simulink model "torqueBalancing2012b"  (Simulink 8.0)
settings: Solver=FixedStepDiscrete  StartTime=0.0  StopTime=CONFIG.SIMULATION_TIME  FixedStep=CONFIG.Ts  RelTol=1e-3
InitFcn:
  | initTorqueBalancing;
values from neighbouring files (symbols this model uses):
  baseToWorldRotationPort = ['/' WBT_modelName '/floatingBaseRotationMatrix:i']    [initTorqueBalancing.m]
  WBT_modelName = 'matlabTorqueBalancing'    [initTorqueBalancing.m]
undefined symbols (not defined in the file or in its folder): bVectorConstraints, CONFIG, ConstraintsMatrix, DiscIntNeverNeededParam, gain, impedencesSat, reg, ROBOT_DOF, ROBOT_DOF_FOR_SIMULINK, sat, SM, sm, Ts
libraries: WBToolboxLibrary x139, simulink x11, WBCLibrary x2
(part 1 of 3)
settings Model: Creator=daniele  LastModifiedBy=gnava
settings DebuggingCC: FcnCallInpInsideContextMsg=EnableAllAsWarning  FrameProcessingCompatibilityMsg=error
settings SFSimCC: SimParseCustomCode=off
settings CodeAppCC: CustomSymbolStrType=$N$R$M_T
settings GRTTargetCC: CodeReplacementLibrary=C89/C90 (ANSI)  CombineOutputUpdateFcns=off  GRTInterface=on

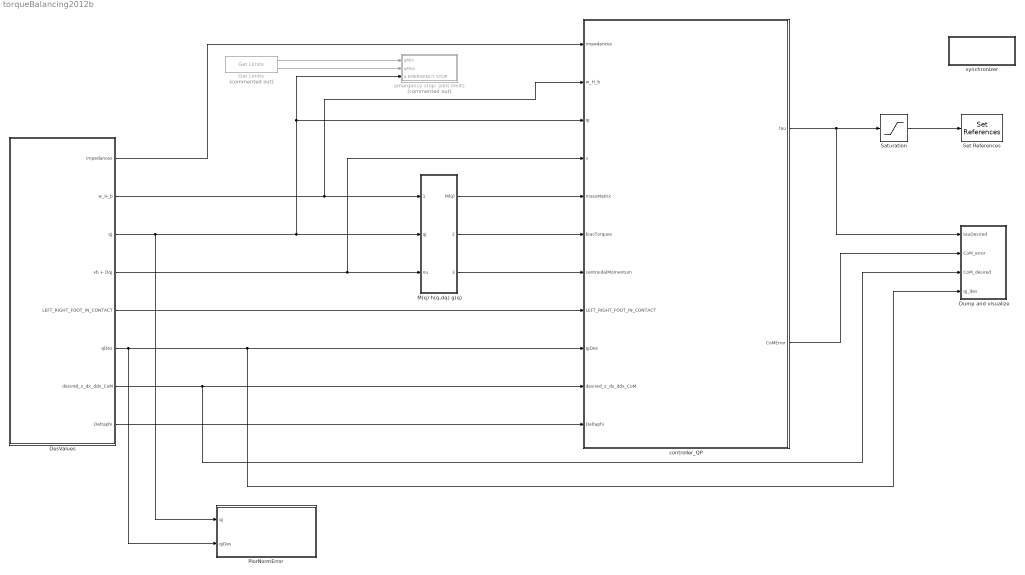
== system torqueBalancing2012b ==
  DesValues : Subsystem  Priority=-10
  Dump and visualize : Subsystem
  Get Limits : WBToolboxLibrary/wholeBodyStates/Get Limits  Commented=on  limitsType=Position  robotName=WBT_robotName  localName=WBT_modelName  wbiFile=WBT_wbiFilename  wbiList=WBT_wbiList
  M(q) h(q,dq) g(q) : Subsystem
  PlorNormError : Subsystem
  Saturation : Saturate  UpperLimit=sat.torque  LowerLimit=-sat.torque
  Set References : WBToolboxLibrary/wholeBodyActuators/Set References  controlType=Torque  robotName=WBT_robotName  localName=WBT_modelName  wbiFile=WBT_wbiFilename  wbiList=WBT_wbiList
  controller_QP : Subsystem
  emergency stop: joint limits : Subsystem  Commented=on
  synchronizer : Subsystem
      mask Display: disp('SYNCHRONIZER')
  wires:
  M(q) h(q,dq) g(q)/1(M(q)) -> controller_QP/5(massMatrix)
  Get Limits/1 -> emergency stop: joint limits/1(qMin)
  Get Limits/2 -> emergency stop: joint limits/2(qMax)
  M(q) h(q,dq) g(q)/2(biasTorques) -> controller_QP/6(biasTorques)
  M(q) h(q,dq) g(q)/3(H(q,dq)) -> controller_QP/7(centroidalMomentum)
  controller_QP/1("tau ") -> Dump and visualize/1(tauDesired), Saturation/1
  controller_QP/2(CoMError) -> Dump and visualize/2(CoM_error)
  DesValues/6(qDes) -> PlorNormError/2(qjDes), controller_QP/9(qjDes), Dump and visualize/4(qj_des)
  DesValues/5(LEFT_RIGHT_FOOT_IN_CONTACT) -> controller_QP/8(LEFT_RIGHT_FOOT_IN_CONTACT)
  DesValues/7(desired_x_dx_ddx_CoM) -> Dump and visualize/3(CoM_desired), controller_QP/10(desired_x_dx_ddx_CoM)
  DesValues/1(impedances) -> controller_QP/1(impedances)
  Saturation/1 -> Set References/1
  DesValues/2(w_H_b) -> controller_QP/2(w_H_b), M(q) h(q,dq) g(q)/1(w_H_b)
  DesValues/4(vb + Dqj) -> controller_QP/4(v), M(q) h(q,dq) g(q)/3(nu)
  DesValues/3(qj) -> PlorNormError/1(qj), emergency stop: joint limits/3(q EMERGENCY STOP), controller_QP/3(qj), M(q) h(q,dq) g(q)/2(qj)
  DesValues/8(Deltaphi) -> controller_QP/11(Deltaphi)

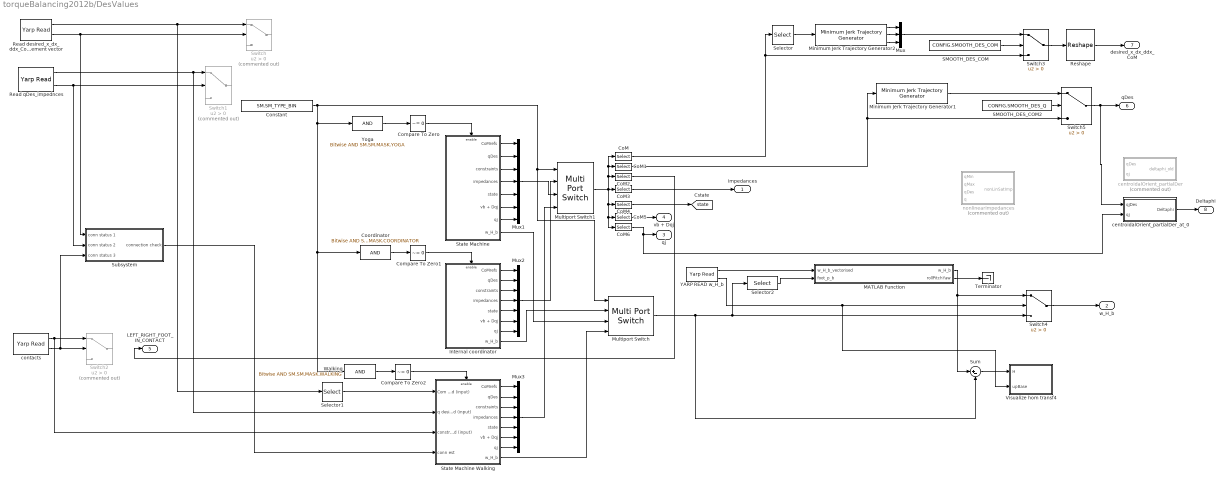
== system torqueBalancing2012b/DesValues ==
  CoM : Selector  InputPortWidth=18+4*ROBOT_DOF  IndexOptions=Index vector (dialog)  Indices=[1:9]  OutputSizes=1
  CoM1 : Selector  InputPortWidth=18+4*ROBOT_DOF  IndexOptions=Index vector (dialog)  Indices=[10:9+ROBOT_DOF]  OutputSizes=1
  CoM2 : Selector  InputPortWidth=18+4*ROBOT_DOF  IndexOptions=Index vector (dialog)  Indices=[10+ROBOT_DOF,11+ROBOT_DOF]  OutputSizes=1
  CoM3 : Selector  InputPortWidth=18+4*ROBOT_DOF  IndexOptions=Index vector (dialog)  Indices=[12+ROBOT_DOF:11+2*ROBOT_DOF]  OutputSizes=1
  CoM4 : Selector  InputPortWidth=18+4*ROBOT_DOF  IndexOptions=Index vector (dialog)  Indices=[12+2*ROBOT_DOF]  OutputSizes=1
  CoM5 : Selector  InputPortWidth=18+4*ROBOT_DOF  IndexOptions=Index vector (dialog)  Indices=[13+2*ROBOT_DOF:18+3*ROBOT_DOF]  OutputSizes=1
  CoM6 : Selector  InputPortWidth=18+4*ROBOT_DOF  IndexOptions=Index vector (dialog)  Indices=[19+3*ROBOT_DOF:18+4*ROBOT_DOF]  OutputSizes=1
  Compare To Zero : simulink/Logic and Bit Operations/Compare To Zero  relop=~=  OutDataTypeStr=boolean
  Compare To Zero1 : simulink/Logic and Bit Operations/Compare To Zero  relop=~=  OutDataTypeStr=boolean
  Compare To Zero2 : simulink/Logic and Bit Operations/Compare To Zero  relop=~=  OutDataTypeStr=boolean
  Constant : Constant  Priority=-10  Value=SM.SM_TYPE_BIN  OutDataTypeStr=uint8
  Coordinator : simulink/Logic and Bit Operations/Bitwise Operator  logicop=AND  UseBitMask=on  BitMask=SM.SM.MASK.COORDINATOR  BitMaskRealWorld=Stored Integer
  Internal coordinator : Subsystem
  MATLAB Function : MATLAB Function  TreatAsAtomicUnit=on
  Minimum Jerk Trajectory Generator1 : WBToolboxLibrary/Utilities/Minimum Jerk Trajectory Generator  externalSettlingTime=off  settlingTime=references.joints.smoothingTime  sampleTime=CONFIG.Ts  firstDerivatives=off  secondDerivatives=off  explicitInitialValue=off
  Minimum Jerk Trajectory Generator2 : WBToolboxLibrary/Utilities/Minimum Jerk Trajectory Generator  externalSettlingTime=off  settlingTime=references.com.smoothingTime  sampleTime=CONFIG.Ts  firstDerivatives=on  secondDerivatives=on  explicitInitialValue=off
  Multiport Switch : MultiPortSwitch  DataPortOrder=Specify indices  DataPortIndices={1, 2, 4}
  Multiport Switch1 : MultiPortSwitch  DataPortOrder=Specify indices  DataPortIndices={1, 2, 4}
  Mux : Mux  Inputs=3
  Mux1 : Mux  Inputs=7
  Mux2 : Mux  Inputs=7
  Mux3 : Mux  Inputs=7
  Read desired_x_dx_ddx_CoM as 9 element vector : WBToolboxLibrary/Utilities/Yarp Read  portName=['/' WBT_modelName '/comDes:i']  signalSize=9  blocking=off  timestamp=off  autoconnect=off  errorOnConnection=on
  Read qDes_impednces : WBToolboxLibrary/Utilities/Yarp Read  portName=['/' WBT_modelName '/qDes:i']  signalSize=ROBOT_DOF  blocking=off  timestamp=off  autoconnect=off  errorOnConnection=on
  Reshape : Reshape  OutputDimensionality=Customize  OutputDimensions=[3,3]
  SMOOTH_DES_COM : Constant  Value=CONFIG.SMOOTH_DES_COM
  SMOOTH_DES_COM2 : Constant  Value=CONFIG.SMOOTH_DES_Q
  Selector : Selector  InputPortWidth=9  IndexOptions=Index vector (dialog)  Indices=[1 2 3]  OutputSizes=1
  Selector1 : Selector  InputPortWidth=9  IndexOptions=Index vector (dialog)  Indices=[1 2 3]  OutputSizes=1
  Selector2 : Selector  NumberOfDimensions=2  InputPortWidth=3  IndexOptions=Index vector (dialog),Index vector (dialog)  Indices=[1 2 3],4  OutputSizes=1,1
  State Machine : Subsystem  Priority=-100
  State Machine Walking : Subsystem  Priority=-100
  Subsystem : Subsystem
  Sum : Sum  Inputs=|+-
  Switch : Switch  Commented=on  Criteria=u2 > Threshold
  Switch1 : Switch  Commented=on  Criteria=u2 > Threshold
  Switch2 : Switch  Commented=on  Criteria=u2 > Threshold
  Switch3 : Switch  Criteria=u2 > Threshold
  Switch4 : Switch  Criteria=u2 > Threshold
  Switch5 : Switch  Criteria=u2 > Threshold
  Terminator : Terminator
  Visualize hom transf4 : Subsystem
  Walking : simulink/Logic and Bit Operations/Bitwise Operator  logicop=AND  UseBitMask=on  BitMask=SM.SM.MASK.WALKING  BitMaskRealWorld=Stored Integer
  YARP READ w_H_b : WBToolboxLibrary/Utilities/Yarp Read  portName=[baseToWorldRotationPort]  signalSize=16  blocking=off  timestamp=off  autoconnect=off  errorOnConnection=on
  Yoga : simulink/Logic and Bit Operations/Bitwise Operator  logicop=AND  UseBitMask=on  BitMask=SM.SM.MASK.YOGA  BitMaskRealWorld=Stored Integer
  centroidalOrient_partialDer : Subsystem  Commented=on
  centroidalOrient_partialDer_at_0 : Subsystem
  contacts : WBToolboxLibrary/Utilities/Yarp Read  portName=['/' WBT_modelName '/constraints:i']  signalSize=2  blocking=off  timestamp=off  autoconnect=off  errorOnConnection=on
  nonlinearImpedances : Subsystem  Commented=on
  impedances : Outport
  w_H_b : Outport  Port=2
  qj : Outport  Port=3
  vb + Dqj : Outport  Port=4
  LEFT_RIGHT_FOOT_IN_CONTACT : Outport  Port=5
  qDes : Outport  Port=6
  desired_x_dx_ddx_CoM : Outport  Port=7
  Deltaphi : Outport  Port=8
  tag scope: state=global
  wires:
  Read desired_x_dx_ddx_CoM as 9 element vector/2 -> Subsystem/1(conn status 1), Switch/2
  Read desired_x_dx_ddx_CoM as 9 element vector/1 -> Selector1/1, Switch/1
  Reshape/1 -> desired_x_dx_ddx_CoM/1
  Read qDes_impednces/2 -> Subsystem/2(conn status 2), Switch1/2
  contacts/2 -> Subsystem/3(conn status 3), Switch2/2
  CoM2/1 -> LEFT_RIGHT_FOOT_IN_CONTACT/1
  CoM/1 -> Selector/1, Switch3/3
  Selector/1 -> Minimum Jerk Trajectory Generator2/1
  Minimum Jerk Trajectory Generator2/1 -> Mux/1
  Minimum Jerk Trajectory Generator2/2 -> Mux/2
  Minimum Jerk Trajectory Generator2/3 -> Mux/3
  Mux/1 -> Switch3/1
  Switch3/1 -> Reshape/1
  SMOOTH_DES_COM/1 -> Switch3/2
  SMOOTH_DES_COM2/1 -> Switch5/2
  CoM1/1 -> Minimum Jerk Trajectory Generator1/1, Switch5/3
  Constant/1 -> Multiport Switch/1, Multiport Switch1/1, Coordinator/1, Walking/1, Yoga/1
  State Machine/3(constraints) -> Mux1/3
  State Machine/2(qDes) -> Mux1/2
  State Machine/1(CoMrefs) -> Mux1/1
  Internal coordinator/1(CoMrefs) -> Mux2/1
  Internal coordinator/2(qDes) -> Mux2/2
  Internal coordinator/3(constraints) -> Mux2/3
  Multiport Switch1/1 -> CoM/1, CoM1/1, CoM2/1, CoM6/1, CoM5/1, CoM4/1, CoM3/1
  CoM3/1 -> impedances/1
  State Machine/4(impedances) -> Mux1/4
  Internal coordinator/4(impedances) -> Mux2/4
  State Machine/5(state) -> Mux1/5
  Internal coordinator/5(state) -> Mux2/5
  CoM4/1 -> [state]
  Internal coordinator/6(vb + Dqj) -> Mux2/6
  Internal coordinator/7(qj) -> Mux2/7
  State Machine/6(vb + Dqj) -> Mux1/6
  State Machine/7(qj) -> Mux1/7
  CoM5/1 -> vb + Dqj/1
  Minimum Jerk Trajectory Generator1/1 -> Switch5/1
  State Machine Walking/4(impedances) -> Mux3/4
  State Machine Walking/3(constraints) -> Mux3/3
  State Machine Walking/5(state) -> Mux3/5
  State Machine Walking/6(vb + Dqj) -> Mux3/6
  State Machine Walking/1(CoMrefs) -> Mux3/1
  State Machine Walking/7(qj) -> Mux3/7
  Coordinator/1 -> Compare To Zero1/1
  Yoga/1 -> Compare To Zero/1
  Walking/1 -> Compare To Zero2/1
  Mux3/1 -> Multiport Switch1/4
  State Machine Walking/8(w_H_b) -> Multiport Switch/4
  Selector1/1 -> State Machine Walking/1(Com desired (input))
  Compare To Zero/1 -> State Machine/Enable
  Compare To Zero1/1 -> Internal coordinator/Enable
  Compare To Zero2/1 -> State Machine Walking/Enable
  Mux1/1 -> Multiport Switch1/3
  Mux2/1 -> Multiport Switch1/2
  State Machine/8(w_H_b) -> Multiport Switch/3
  Internal coordinator/8(w_H_b) -> Multiport Switch/2
  Read qDes_impednces/1 -> State Machine Walking/2(q desired (input)), Switch1/1
  Subsystem/1(connection check) -> State Machine Walking/4(conn est)
  State Machine Walking/2(qDes) -> Mux3/2
  contacts/1 -> State Machine Walking/3(constraints desired (input)), Switch2/1
  YARP READ w_H_b/1 -> MATLAB Function/1(w_H_b_vectorised)
  MATLAB Function/1(w_H_b) -> Sum/1, Switch4/1
  Selector2/1 -> MATLAB Function/2(foot_p_b)
  Sum/1 -> Visualize hom transf4/1(H)
  Switch4/1 -> w_H_b/1
  Multiport Switch/1 -> Selector2/1, Switch4/3, Sum/2
  YARP READ w_H_b/2 -> Switch4/2, Visualize hom transf4/2(upBase)
  MATLAB Function/2(rollPitchYaw) -> Terminator/1
  Switch5/1 -> centroidalOrient_partialDer_at_0/1(qjDes), qDes/1
  CoM6/1 -> centroidalOrient_partialDer_at_0/2(qj), qj/1
  centroidalOrient_partialDer_at_0/1(Deltaphi) -> Deltaphi/1

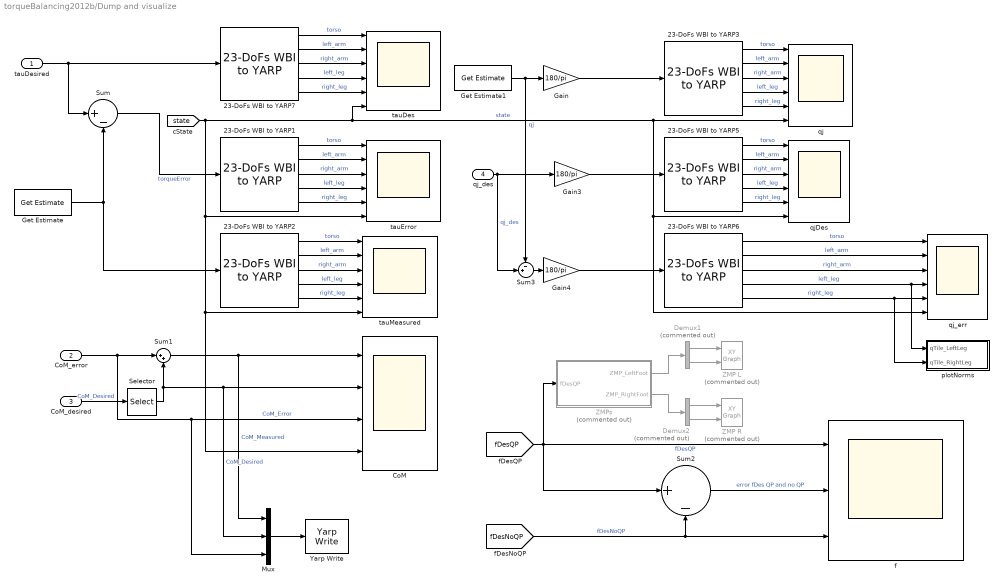
== system torqueBalancing2012b/Dump and visualize ==
  tauDesired : Inport
  CoM_error : Inport  Port=2
  CoM_desired : Inport  Port=3
  qj_des : Inport  Port=4
  23-DoFs WBI to YARP{1..3,5..7} (6 alike) : WBToolboxLibrary/Utilities/23-DoFs WBI to YARP
  CoM : Scope  NumInputPorts=4
      settings: ShowLegends=on  TimeRange=400  YMin=-0.22651~-0.2206~-0.01616~-0.125  YMax=0.64756~0.64126~0.01985~11.125  SaveName=CoM_data
  Demux1 : Demux  Commented=on  Outputs=2
  Demux2 : Demux  Commented=on  Outputs=2
  Gain : Gain  Gain=180/pi
  Gain3 : Gain  Gain=180/pi
  Gain4 : Gain  Gain=180/pi
  Get Estimate : WBToolboxLibrary/wholeBodyStates/Get Estimate  estimateType=Joints Torque  robotName=WBT_robotName  localName=WBT_modelName  wbiFile=WBT_wbiFilename  wbiList=WBT_wbiList
  Get Estimate1 : WBToolboxLibrary/wholeBodyStates/Get Estimate  estimateType=Joints Position  robotName=WBT_robotName  localName=WBT_modelName  wbiFile=WBT_wbiFilename  wbiList=WBT_wbiList
  Mux : Mux  Inputs=3
  Selector : Selector  NumberOfDimensions=2  IndexOptions=Index vector (dialog),Index vector (dialog)  Indices=[1:3],1  OutputSizes=1,1
  Sum : Sum  Inputs=|+-
  Sum1 : Sum  Inputs=|++
  Sum2 : Sum  Inputs=|+-
  Sum3 : Sum  Inputs=-+|
  Yarp Write : WBToolboxLibrary/Utilities/Yarp Write  portName='/oneFootBalancing/comInfo:o'  autoconnect=off  errorOnConnection=on
  ZMP L : simulink/Sinks/XY Graph  Commented=on  xmin=gain.footSize(1,1)  xmax=gain.footSize(1,2)  ymin=gain.footSize(2,1)  ymax=gain.footSize(2,2)  st=-1
  ZMP R : simulink/Sinks/XY Graph  Commented=on  xmin=gain.footSize(1,1)  xmax=gain.footSize(1,2)  ymin=gain.footSize(2,1)  ymax=gain.footSize(2,2)  st=-1
  ZMPs : Subsystem  Commented=on
  f : Scope  NumInputPorts=3
      settings: TimeRange=40  YMin=-57.20094~-0.00771~-57.19974  YMax=249.13374~0.00771~249.13391  SaveName=ScopeData2
  plotNorms : Subsystem
  qj : Scope  NumInputPorts=6
      settings: ShowLegends=on  TimeRange=40  YMin=-32.23366~-73.47113~-76.53021~-115.83931~-22.69232~-0.125  YMax=12.59592~104.84995~80.45225~96.1311~29.20641~11.125  SaveName=qj_and_v
  qjDes : Scope  NumInputPorts=6
      settings: ShowLegends=on  TimeRange=40  YMin=-3.5~-40~-40~-15~-10~2  YMax=0.5~50~50~15~12.5~2  SaveName=qj_and_v3
  qj_err : Scope  NumInputPorts=6
      settings: ShowLegends=on  TimeRange=40  YMin=-5~-3~-2~-7.5~-3~2  YMax=3~4~3.5~7.5~6~2  SaveName=qj_and_v4
  tauDes : Scope  NumInputPorts=6
      settings: ShowLegends=on  TimeRange=14  YMin=-58.64434~-21.39097~-21.52762~-81.43596~-94.54214~0.625  YMax=46.53013~21.42382~22.63023~161.15223~80.75083~4.375  SaveName=tauDes
  tauError : Scope  NumInputPorts=6
      settings: ShowLegends=on  TimeRange=90  YMin=-2.6459~-3.11955~-3.43578~-20.45507~-6.22161~0.625  YMax=3.57267~4.34787~4.22527~21.32013~5.56801~4.375  SaveName=tauError
  tauMeasured : Scope  NumInputPorts=6
      settings: ShowLegends=on  TimeRange=14  YMin=-7~-2.5~-2.5~-3~-4~2  YMax=0~1.5~1.5~2~3~2  SaveName=tauMeasured
  wires:
  CoM_error/1 -> Sum1/1, Mux/3, CoM/3  "CoM_Error"
  CoM_desired/1 -> Selector/1  "CoM_Desired"
  Sum1/1 -> Mux/1, CoM/1  "CoM_Measured"
  Get Estimate1/1 -> Sum3/1, Gain/1  "qj"
  Gain/1 -> 23-DoFs WBI to YARP3/1
  23-DoFs WBI to YARP3/5 -> qj/5  "right_leg"
  23-DoFs WBI to YARP3/1 -> qj/1  "torso"
  23-DoFs WBI to YARP3/2 -> qj/2  "left_arm"
  23-DoFs WBI to YARP3/4 -> qj/4  "left_leg"
  23-DoFs WBI to YARP3/3 -> qj/3  "right_arm"
  [fDesQP] -> ZMPs/1(fDesQP), Sum2/1, f/1  "fDesQP"
  ZMPs/1(ZMP_LeftFoot) -> Demux1/1
  ZMPs/2(ZMP_RightFoot) -> Demux2/1
  Demux1/1 -> ZMP L/1
  Demux1/2 -> ZMP L/2
  Demux2/1 -> ZMP R/1
  Demux2/2 -> ZMP R/2
  Sum2/1 -> f/2  "error fDes QP and no QP"
  [fDesNoQP] -> Sum2/2, f/3  "fDesNoQP"
  tauDesired/1 -> 23-DoFs WBI to YARP7/1, Sum/1
  Get Estimate/1 -> 23-DoFs WBI to YARP2/1, Sum/2
  23-DoFs WBI to YARP7/5 -> tauDes/5  "right_leg"
  23-DoFs WBI to YARP7/1 -> tauDes/1  "torso"
  23-DoFs WBI to YARP7/2 -> tauDes/2  "left_arm"
  23-DoFs WBI to YARP7/4 -> tauDes/4  "left_leg"
  23-DoFs WBI to YARP7/3 -> tauDes/3  "right_arm"
  23-DoFs WBI to YARP1/5 -> tauError/5  "right_leg"
  23-DoFs WBI to YARP1/1 -> tauError/1  "torso"
  23-DoFs WBI to YARP1/2 -> tauError/2  "left_arm"
  23-DoFs WBI to YARP1/4 -> tauError/4  "left_leg"
  23-DoFs WBI to YARP1/3 -> tauError/3  "right_arm"
  Sum/1 -> 23-DoFs WBI to YARP1/1  "torqueError"
  23-DoFs WBI to YARP2/5 -> tauMeasured/5  "right_leg"
  23-DoFs WBI to YARP2/1 -> tauMeasured/1  "torso"
  23-DoFs WBI to YARP2/2 -> tauMeasured/2  "left_arm"
  23-DoFs WBI to YARP2/4 -> tauMeasured/4  "left_leg"
  23-DoFs WBI to YARP2/3 -> tauMeasured/3  "right_arm"
  qj_des/1 -> Sum3/2, Gain3/1  "qj_des"
  Gain3/1 -> 23-DoFs WBI to YARP5/1
  23-DoFs WBI to YARP5/5 -> qjDes/5  "right_leg"
  23-DoFs WBI to YARP5/1 -> qjDes/1  "torso"
  23-DoFs WBI to YARP5/2 -> qjDes/2  "left_arm"
  23-DoFs WBI to YARP5/4 -> qjDes/4  "left_leg"
  23-DoFs WBI to YARP5/3 -> qjDes/3  "right_arm"
  Gain4/1 -> 23-DoFs WBI to YARP6/1
  23-DoFs WBI to YARP6/5 -> plotNorms/2(qTile_RightLeg), qj_err/5  "right_leg"
  23-DoFs WBI to YARP6/1 -> qj_err/1  "torso"
  23-DoFs WBI to YARP6/2 -> qj_err/2  "left_arm"
  23-DoFs WBI to YARP6/4 -> plotNorms/1(qTile_LeftLeg), qj_err/4  "left_leg"
  23-DoFs WBI to YARP6/3 -> qj_err/3  "right_arm"
  Sum3/1 -> Gain4/1
  Selector/1 -> Sum1/2, Mux/2, CoM/2  "CoM_Desired"
  [state] -> tauDes/6, qj_err/6, qjDes/6, qj/6, CoM/4, tauMeasured/6, tauError/6  "state"
  Mux/1 -> Yarp Write/1

== system torqueBalancing2012b/M(q) h(q,dq) g(q) ==
  w_H_b : Inport
  qj : Inport  Port=2
  nu : Inport  Port=3
  Centroidal Momentum : WBToolboxLibrary/wholeBodyModel/Dynamics/Centroidal Momentum  robotName=WBT_robotName  localName=WBT_modelName  wbiFile=WBT_wbiFilename  wbiList=WBT_wbiList
  "CoM6D ->  CoMXYZ1" : Selector  InputPortWidth=6+ROBOT_DOF  IndexOptions=Index vector (dialog)  Indices=[7:6+ROBOT_DOF]  OutputSizes=1
  "CoM6D ->  CoMXYZ2" : Selector  InputPortWidth=6+ROBOT_DOF  IndexOptions=Index vector (dialog)  Indices=[1 2 3 4 5 6]  OutputSizes=1
  Get Bias Forces : WBToolboxLibrary/wholeBodyModel/Dynamics/Get Bias Forces  robotName=WBT_robotName  localName=WBT_modelName  wbiFile=WBT_wbiFilename  wbiList=WBT_wbiList
  Mass Matrix : WBToolboxLibrary/wholeBodyModel/Dynamics/Mass Matrix  robotName=WBT_robotName  localName=WBT_modelName  wbiFile=WBT_wbiFilename  wbiList=WBT_wbiList
  M(q) : Outport
  biasTorques : Outport  Port=2
  H(q,dq) : Outport  Port=3
  wires:
  Mass Matrix/1 -> M(q)/1
  Centroidal Momentum/1 -> H(q,dq)/1
  Get Bias Forces/1 -> biasTorques/1
  w_H_b/1 -> Centroidal Momentum/1, Get Bias Forces/1, Mass Matrix/1
  qj/1 -> Centroidal Momentum/2, Get Bias Forces/2, Mass Matrix/2
  "CoM6D ->  CoMXYZ2"/1 -> Centroidal Momentum/3, Get Bias Forces/3
  "CoM6D ->  CoMXYZ1"/1 -> Get Bias Forces/4, Centroidal Momentum/4
  nu/1 -> "CoM6D ->  CoMXYZ1"/1, "CoM6D ->  CoMXYZ2"/1

== system torqueBalancing2012b/PlorNormError ==
  qj : Inport
  qjDes : Inport  Port=2
  Dot Product : DotProduct  InputSameDT=on  OutDataTypeStr=Inherit: Inherit via internal rule
  PosNorm : Scope
      settings: TimeRange=120  YMin=1.735  YMax=1.76  SaveName=ScopeData4
  Sqrt : Sqrt  SaturateOnIntegerOverflow=on
  Sum : Sum  Inputs=|-+
  wires:
  qj/1 -> Sum/2
  qjDes/1 -> Sum/1
  Sum/1 -> Dot Product/1, Dot Product/2
  Dot Product/1 -> Sqrt/1
  Sqrt/1 -> PosNorm/1

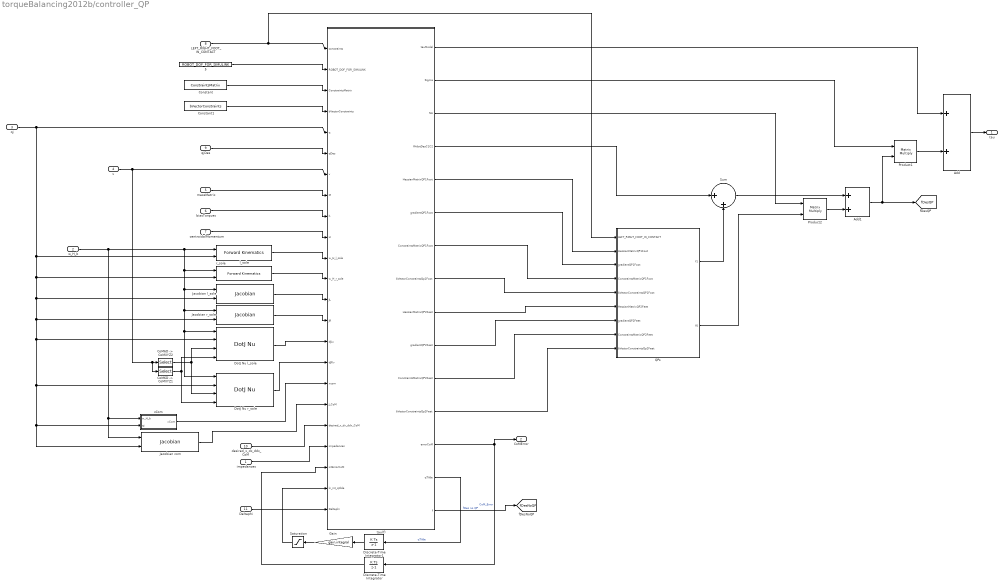
== system torqueBalancing2012b/controller_QP ==
  impedances : Inport
  w_H_b : Inport  Port=2
  qj : Inport  Port=3
  v : Inport  Port=4
  massMatrix : Inport  Port=5
  biasTorques : Inport  Port=6
  centroidalMomentum : Inport  Port=7
  LEFT_RIGHT_FOOT_IN_CONTACT : Inport  Port=8
  qjDes : Inport  Port=9
  desired_x_dx_ddx_CoM : Inport  Port=10
  Deltaphi : Inport  Port=11
  "    5" : Constant  Value=ROBOT_DOF_FOR_SIMULINK
  Add : Sum
  Add1 : Sum
  "CoM6D ->  CoMXYZ1" : Selector  InputPortWidth=6+ROBOT_DOF  IndexOptions=Index vector (dialog)  Indices=[7:6+ROBOT_DOF]  OutputSizes=1
  "CoM6D ->  CoMXYZ2" : Selector  InputPortWidth=6+ROBOT_DOF  IndexOptions=Index vector (dialog)  Indices=[1 2 3 4 5 6]  OutputSizes=1
  Constant : Constant  Value=ConstraintsMatrix
  Constant1 : Constant  Value=bVectorConstraints
  Discrete-Time Integrator : DiscreteIntegrator  InitialCondition=[0 0 0]  SampleTime=CONFIG.Ts  ICPrevOutput=DiscIntNeverNeededParam  ICPrevScaledInput=DiscIntNeverNeededParam
  Discrete-Time Integrator1 : DiscreteIntegrator  InitialCondition=zeros(ROBOT_DOF,1)  SampleTime=CONFIG.Ts  ICPrevOutput=DiscIntNeverNeededParam  ICPrevScaledInput=DiscIntNeverNeededParam
  "DotJ Nu l_sole " : WBToolboxLibrary/wholeBodyModel/Jacobians/DotJ Nu  frameName='l_sole'  robotName=WBT_robotName  localName=WBT_modelName  wbiFile=WBT_wbiFilename  wbiList=WBT_wbiList
  "DotJ Nu r_sole " : WBToolboxLibrary/wholeBodyModel/Jacobians/DotJ Nu  frameName='r_sole'  robotName=WBT_robotName  localName=WBT_modelName  wbiFile=WBT_wbiFilename  wbiList=WBT_wbiList
  Gain : Gain  Gain=gain.integral
  Jacobian com : WBToolboxLibrary/wholeBodyModel/Jacobians/Jacobian  frameName='com'  robotName=WBT_robotName  localName=WBT_modelName  wbiFile=WBT_wbiFilename  wbiList=WBT_wbiList
  Jacobian l_sole : WBToolboxLibrary/wholeBodyModel/Jacobians/Jacobian  frameName='l_sole'  robotName=WBT_robotName  localName=WBT_modelName  wbiFile=WBT_wbiFilename  wbiList=WBT_wbiList
  Jacobian r_sole : WBToolboxLibrary/wholeBodyModel/Jacobians/Jacobian  frameName='r_sole'  robotName=WBT_robotName  localName=WBT_modelName  wbiFile=WBT_wbiFilename  wbiList=WBT_wbiList
  Product1 : Product  Multiplication=Matrix(*)
  Product2 : Product  Multiplication=Matrix(*)
  QPs : Subsystem
  Saturation : Saturate  UpperLimit=sat.integral  LowerLimit=-sat.integral
  Sum : Sum  Inputs=|++
  l_sole : WBToolboxLibrary/wholeBodyModel/Kinematics/Forward Kinematics  frameName='l_sole'  robotName=WBT_robotName  localName=WBT_modelName  wbiFile=WBT_wbiFilename  wbiList=WBT_wbiList
  r_sole : WBToolboxLibrary/wholeBodyModel/Kinematics/Forward Kinematics  frameName='r_sole'  robotName=WBT_robotName  localName=WBT_modelName  wbiFile=WBT_wbiFilename  wbiList=WBT_wbiList
  "tau(f) " : MATLAB Function  TreatAsAtomicUnit=on
  xCom : Subsystem
  "tau " : Outport
  CoMError : Outport  Port=2
  tag scope: fDesNoQP=global, fDesQP=global
  wires:
  LEFT_RIGHT_FOOT_IN_CONTACT/1 -> QPs/1(LEFT_RIGHT_FOOT_IN_CONTACT), "tau(f) "/1(constraints)
  Discrete-Time Integrator/1 -> "tau(f) "/21(intErrorCoM)
  "tau(f) "/13(errorCoM) -> CoMError/1, Discrete-Time Integrator/1  "CoM_Error"
  Discrete-Time Integrator1/1 -> Gain/1
  "tau(f) "/14(qTilde) -> Discrete-Time Integrator1/1  "qTilde"
  Gain/1 -> Saturation/1
  Saturation/1 -> "tau(f) "/22(ki_int_qtilde)
  qj/1 -> xCom/2(qj), Jacobian com/2, "DotJ Nu r_sole "/2, "DotJ Nu l_sole "/2, Jacobian r_sole/2, Jacobian l_sole/2, r_sole/2, l_sole/2, "tau(f) "/5(q)
  qjDes/1 -> "tau(f) "/6(qDes)
  massMatrix/1 -> "tau(f) "/8(M)
  biasTorques/1 -> "tau(f) "/9(h)
  desired_x_dx_ddx_CoM/1 -> "tau(f) "/19(desired_x_dx_ddx_CoM)
  impedances/1 -> "tau(f) "/20(impedances)
  centroidalMomentum/1 -> "tau(f) "/10(H)
  r_sole/1 -> "tau(f) "/12(w_H_r_sole)
  l_sole/1 -> "tau(f) "/11(w_H_l_sole)
  Jacobian l_sole/1 -> "tau(f) "/13(JL)
  Jacobian r_sole/1 -> "tau(f) "/14(JR)
  Jacobian com/1 -> "tau(f) "/18(J_CoM)
  "tau(f) "/5(HessianMatrixQP1Foot) -> QPs/2(HessianMatrixQP1Foot)
  "tau(f) "/6(gradientQP1Foot) -> QPs/3(gradientQP1Foot)
  "tau(f) "/9(HessianMatrixQP2Feet) -> QPs/6(HessianMatrixQP2Feet)
  "tau(f) "/10(gradientQP2Feet) -> QPs/7(gradientQP2Feet)
  "tau(f) "/11(ConstraintsMatrixQP2Feet) -> QPs/8(ConstraintsMatrixQP2Feet)
  "tau(f) "/12(bVectorConstraintsQp2Feet) -> QPs/9(bVectorConstraintsQp2Feet)
  "tau(f) "/4(fHdotDesC1C2) -> Sum/1
  QPs/1(f1) -> Sum/2
  Product1/1 -> Add/2
  "tau(f) "/1(tauModel) -> Add/1
  Add/1 -> "tau "/1
  Add1/1 -> [fDesQP], Product1/2
  "    5"/1 -> "tau(f) "/2(ROBOT_DOF_FOR_SIMULINK)
  Constant/1 -> "tau(f) "/3(ConstraintsMatrix)
  Constant1/1 -> "tau(f) "/4(bVectorConstraints)
  "tau(f) "/7(ConstraintsMatrixQP1Foot) -> QPs/4(ConstraintsMatrixQP1Foot)
  "tau(f) "/8(bVectorConstraintsQp1Foot) -> QPs/5(bVectorConstraintsQP1Foot)
  Sum/1 -> Add1/1
  Product2/1 -> Add1/2
  "tau(f) "/3(NA) -> Product2/1
  "tau(f) "/2(Sigma) -> Product1/1
  "tau(f) "/15(f) -> [fDesNoQP]  "fDes no QP"
  "DotJ Nu l_sole "/1 -> "tau(f) "/15(dJLv)
  "DotJ Nu r_sole "/1 -> "tau(f) "/16(dJRv)
  xCom/1(xCom) -> "tau(f) "/17(xcom)
  v/1 -> "tau(f) "/7(v), "CoM6D ->  CoMXYZ1"/1, "CoM6D ->  CoMXYZ2"/1
  "CoM6D ->  CoMXYZ2"/1 -> "DotJ Nu r_sole "/3, "DotJ Nu l_sole "/3
  "CoM6D ->  CoMXYZ1"/1 -> "DotJ Nu r_sole "/4, "DotJ Nu l_sole "/4
  w_H_b/1 -> xCom/1(w_H_b), Jacobian com/1, "DotJ Nu r_sole "/1, "DotJ Nu l_sole "/1, Jacobian r_sole/1, Jacobian l_sole/1, r_sole/1, l_sole/1
  QPs/2(f0) -> Product2/2
  Deltaphi/1 -> "tau(f) "/23(Deltaphi)

== system torqueBalancing2012b/emergency stop: joint limits ==
  qMin : Inport
  qMax : Inport  Port=2
  q EMERGENCY STOP : Inport  Port=3
  Assertion : Assertion  Enabled=on
  MATLAB Function : MATLAB Function  TreatAsAtomicUnit=on
  index1 : Constant  Value=0.01  VectorParams1D=off
  wires:
  qMin/1 -> MATLAB Function/1(umin)
  qMax/1 -> MATLAB Function/2(umax)
  index1/1 -> MATLAB Function/4(tol)
  q EMERGENCY STOP/1 -> MATLAB Function/3(u)
  MATLAB Function/1(inRange) -> Assertion/1

== system torqueBalancing2012b/synchronizer ==
  GAZEBO_SYNCHRONIZER : Subsystem
  Logical Operator : Logic  Operator=NOT  AllPortsSameDT=off  OutDataTypeStr=boolean
  "ON_GAZEBO " : Constant  Value=CONFIG.ON_GAZEBO
  REAL_TIME_SYNC : Subsystem  Commented=on
  wires:
  Logical Operator/1 -> REAL_TIME_SYNC/Enable
  "ON_GAZEBO "/1 -> GAZEBO_SYNCHRONIZER/Enable, Logical Operator/1

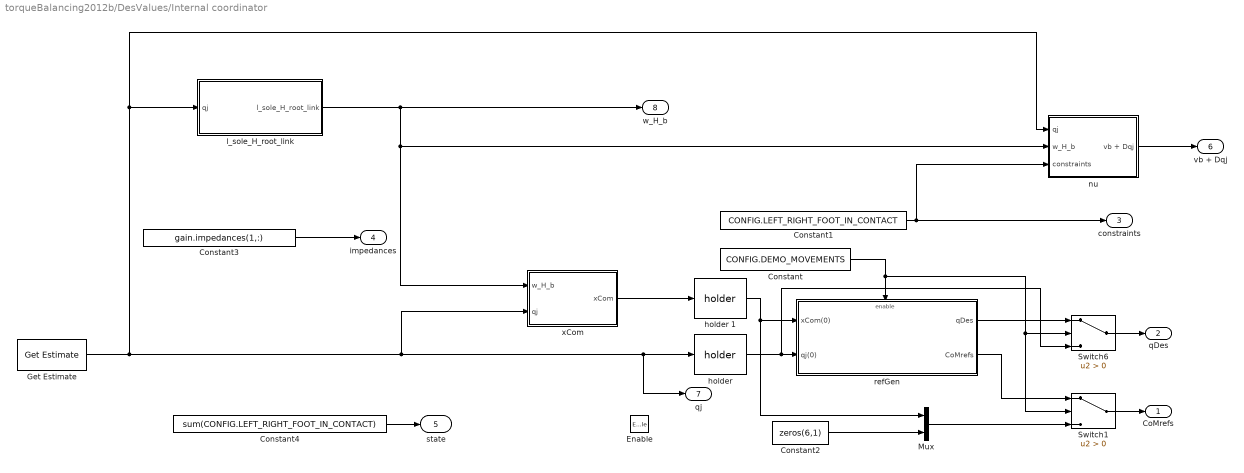
== system torqueBalancing2012b/DesValues/Internal coordinator ==
  Enable : EnablePort
  Constant : Constant  Value=CONFIG.DEMO_MOVEMENTS
  Constant1 : Constant  Value=CONFIG.LEFT_RIGHT_FOOT_IN_CONTACT
  Constant2 : Constant  Value=zeros(6,1)
  Constant3 : Constant  Value=gain.impedances(1,:)
  Constant4 : Constant  Value=sum(CONFIG.LEFT_RIGHT_FOOT_IN_CONTACT)
  Get Estimate : WBToolboxLibrary/wholeBodyStates/Get Estimate  estimateType=Joints Position  robotName=WBT_robotName  localName=WBT_modelName  wbiFile=WBT_wbiFilename  wbiList=WBT_wbiList
  Mux : Mux  Inputs=2
  Switch1 : Switch  Criteria=u2 > Threshold
  Switch6 : Switch  Criteria=u2 > Threshold
  "holder " : WBToolboxLibrary/Utilities/holder 
  holder 1 : WBToolboxLibrary/Utilities/holder 
  l_sole_H_root_link : Subsystem
  nu : Subsystem
  refGen : Subsystem
  xCom : Subsystem
  CoMrefs : Outport
  qDes : Outport  Port=2
  constraints : Outport  Port=3
  impedances : Outport  Port=4
  state : Outport  Port=5
  vb + Dqj : Outport  Port=6
  qj : Outport  Port=7
  w_H_b : Outport  Port=8
  wires:
  Constant1/1 -> nu/3("constraints "), constraints/1
  Get Estimate/1 -> l_sole_H_root_link/1(qj), nu/1(qj), xCom/2(qj), "holder "/1, qj/1
  "holder "/1 -> Switch6/3, refGen/2(qj(0))
  Constant/1 -> Switch1/2, Switch6/2, refGen/Enable
  Switch6/1 -> qDes/1
  Switch1/1 -> CoMrefs/1
  refGen/1(qDes) -> Switch6/1
  refGen/2(CoMrefs) -> Switch1/1
  Mux/1 -> Switch1/3
  Constant2/1 -> Mux/2
  Constant3/1 -> impedances/1
  Constant4/1 -> state/1
  nu/1(vb + Dqj) -> vb + Dqj/1
  holder 1/1 -> Mux/1, refGen/1(xCom(0))
  l_sole_H_root_link/1(l_sole_H_root_link) -> nu/2(w_H_b), xCom/1(w_H_b), w_H_b/1
  xCom/1(xCom) -> holder 1/1

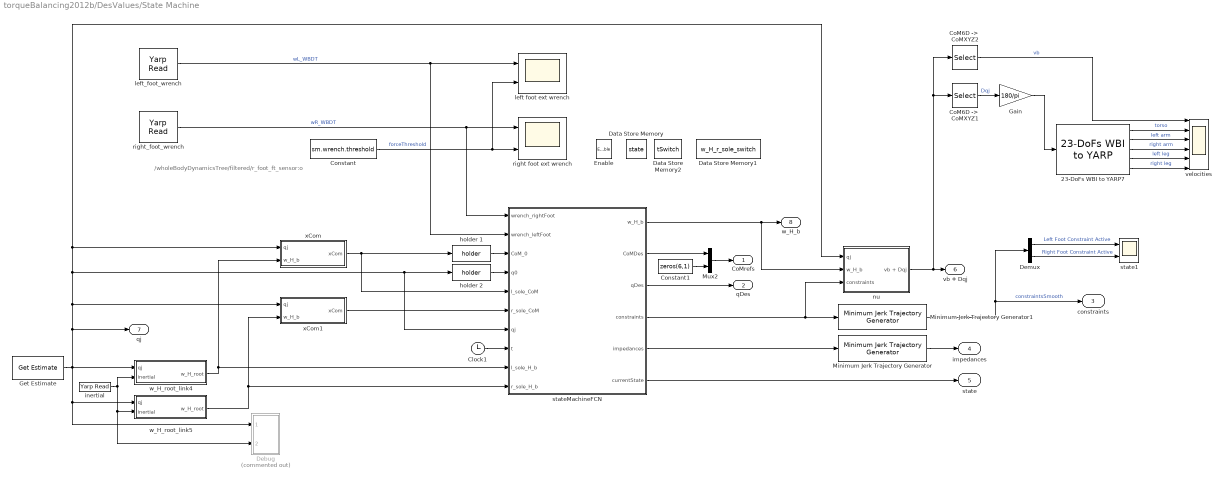
== system torqueBalancing2012b/DesValues/State Machine ==
  note: /wholeBodyDynamicsTree/filtered/r_foot_ft_sensor:o
  Enable : EnablePort
  23-DoFs WBI to YARP7 : WBToolboxLibrary/Utilities/23-DoFs WBI to YARP
  Clock1 : Clock
  "CoM6D ->  CoMXYZ1" : Selector  InputPortWidth=ROBOT_DOF+6  IndexOptions=Index vector (dialog)  Indices=[7:ROBOT_DOF+6]  OutputSizes=1
  "CoM6D ->  CoMXYZ2" : Selector  InputPortWidth=ROBOT_DOF+6  IndexOptions=Index vector (dialog)  Indices=[1 2 3 4 5 6]  OutputSizes=1
  Constant : Constant  Value=sm.wrench.threshold
  Constant1 : Constant  Value=zeros(6,1)
  Data Store Memory : DataStoreMemory  DataStoreName=state  InitialValue=sm.stateAt0  OutDataTypeStr=double
  Data Store Memory1 : DataStoreMemory  DataStoreName=w_H_r_sole_switch  InitialValue=zeros(4)  OutDataTypeStr=double
  Data Store Memory2 : DataStoreMemory  DataStoreName=tSwitch  OutDataTypeStr=double
  Debug : Subsystem  Commented=on
  Demux : Demux  Outputs=2
  Gain : Gain  Gain=180/pi
  Get Estimate : WBToolboxLibrary/wholeBodyStates/Get Estimate  estimateType=Joints Position  robotName=WBT_robotName  localName=WBT_modelName  wbiFile=WBT_wbiFilename  wbiList=WBT_wbiList
  Minimum Jerk Trajectory Generator : WBToolboxLibrary/Utilities/Minimum Jerk Trajectory Generator  externalSettlingTime=off  settlingTime=gain.SmoothingTimeImp  sampleTime=CONFIG.Ts  firstDerivatives=off  secondDerivatives=off  explicitInitialValue=off
  Minimum Jerk Trajectory Generator1 : WBToolboxLibrary/Utilities/Minimum Jerk Trajectory Generator  externalSettlingTime=off  settlingTime=smoothingTimeTransitionDynamics  sampleTime=CONFIG.Ts  firstDerivatives=off  secondDerivatives=off  explicitInitialValue=off
  Mux2 : Mux  Inputs=2
  holder 1 : WBToolboxLibrary/Utilities/holder 
  holder 2 : WBToolboxLibrary/Utilities/holder 
  inertial : WBToolboxLibrary/Utilities/Yarp Read  portName='/icub/inertial'  signalSize=12  blocking=off  timestamp=off  autoconnect=on  errorOnConnection=off
  left foot ext wrench : Scope  NumInputPorts=2
      settings: YMin=-45.83624~-5  YMax=78.73106~5
  left_foot_wrench : WBToolboxLibrary/Utilities/Yarp Read  portName='/wholeBodyDynamicsTree/left_leg/cartesianEndEffectorWrench:o'  signalSize=6  blocking=off  timestamp=off  autoconnect=on  errorOnConnection=off
  nu : Subsystem
  right foot ext wrench : Scope  NumInputPorts=2
      settings: ShowLegends=on  TimeRange=42.68  YMin=-145.04201~-5  YMax=387.7556~5
  right_foot_wrench : WBToolboxLibrary/Utilities/Yarp Read  portName='/wholeBodyDynamicsTree/right_leg/cartesianEndEffectorWrench:o'  signalSize=6  blocking=off  timestamp=off  autoconnect=on  errorOnConnection=off
  state1 : Scope  NumInputPorts=2
      settings: YMin=-0.14635~-5  YMax=1.12737~5  SaveName=ScopeData2
  stateMachineFCN : MATLAB Function  TreatAsAtomicUnit=on
  velocities : Scope  NumInputPorts=6
      settings: YMin=-2.14738~-167.8498~-240.80577~-214.40022~-170.94682~-166.50539  YMax=2.60944~145.16937~76.88393~295.56172~218.42933~230.10458  SaveName=ScopeData2
  w_H_root_link4 : Subsystem  mask{link_name='l_sole'}
      mask prompts: link_name "link name"
      mask help:
      | This block evaluates the homogeneous transformation between the world and the root link, i.e. ^wH_b. It assumes that the link specified by the variable 'link_name' has a constant position
      | w.r.t. an inertial frame, but it can rotate arbitrarily. This rotation is retrived from the IMU sensor.
      mask Display:
      | str = strrep(link_name, '_','\_');
      | port_label('output',1,['{}^{',str '}H_{root}'],'texmode','on')
      | clear str;
      | 
      | port_label('input',1,'q_j','texmode','on')
      | 
      | port_label('input',2,'inertial','texmode','on')
  w_H_root_link5 : Subsystem  mask{link_name='r_sole'}
      mask prompts: link_name "link name"
      mask help:
      | This block evaluates the homogeneous transformation between the world and the root link, i.e. ^wH_b. It assumes that the link specified by the variable 'link_name' has a constant position
      | w.r.t. an inertial frame, but it can rotate arbitrarily. This rotation is retrived from the IMU sensor.
      mask Display:
      | str = strrep(link_name, '_','\_');
      | port_label('output',1,['{}^{',str '}H_{root}'],'texmode','on')
      | clear str;
      | 
      | port_label('input',1,'q_j','texmode','on')
      | 
      | port_label('input',2,'inertial','texmode','on')
  xCom : Subsystem
  xCom1 : Subsystem
  CoMrefs : Outport
  qDes : Outport  Port=2
  constraints : Outport  Port=3
  impedances : Outport  Port=4
  state : Outport  Port=5
  vb + Dqj : Outport  Port=6
  qj : Outport  Port=7
  w_H_b : Outport  Port=8
  wires:
  Constant/1 -> left foot ext wrench/2, right foot ext wrench/2  "forceThreshold"
  right_foot_wrench/1 -> right foot ext wrench/1, stateMachineFCN/1(wrench_rightFoot)  "wR_WBDT"
  xCom/1(xCom) -> stateMachineFCN/5(l_sole_CoM), holder 1/1
  holder 1/1 -> stateMachineFCN/3(CoM_0)
  holder 2/1 -> stateMachineFCN/4(q0)
  Clock1/1 -> stateMachineFCN/8(t)
  stateMachineFCN/3(qDes) -> qDes/1
  stateMachineFCN/2(CoMDes) -> Mux2/1
  Mux2/1 -> CoMrefs/1
  Constant1/1 -> Mux2/2
  stateMachineFCN/5(impedances) -> Minimum Jerk Trajectory Generator/1
  stateMachineFCN/6(currentState) -> state/1
  Minimum Jerk Trajectory Generator1/1 -> Demux/1, constraints/1  "constraintsSmooth"
  stateMachineFCN/4(constraints) -> Minimum Jerk Trajectory Generator1/1, nu/3("constraints ")
  Demux/1 -> state1/1  "Left Foot Constraint Active"
  Demux/2 -> state1/2  "Right Foot Constraint Active"
  left_foot_wrench/1 -> stateMachineFCN/2(wrench_leftFoot), left foot ext wrench/1  "wL_WBDT"
  stateMachineFCN/1(w_H_b) -> nu/2(w_H_b), w_H_b/1
  xCom1/1(xCom) -> stateMachineFCN/6(r_sole_CoM)
  nu/1(vb + Dqj) -> "CoM6D ->  CoMXYZ1"/1, "CoM6D ->  CoMXYZ2"/1, vb + Dqj/1
  Minimum Jerk Trajectory Generator/1 -> impedances/1
  "CoM6D ->  CoMXYZ2"/1 -> velocities/1  "vb"
  "CoM6D ->  CoMXYZ1"/1 -> Gain/1  "Dqj"
  23-DoFs WBI to YARP7/1 -> velocities/2  "torso"
  23-DoFs WBI to YARP7/2 -> velocities/3  "left arm"
  23-DoFs WBI to YARP7/3 -> velocities/4  "right arm"
  23-DoFs WBI to YARP7/4 -> velocities/5  "left leg"
  23-DoFs WBI to YARP7/5 -> velocities/6  "right leg"
  Gain/1 -> 23-DoFs WBI to YARP7/1
  w_H_root_link4/1(w_H_root) -> stateMachineFCN/9(l_sole_H_b), xCom/2(w_H_b)
  w_H_root_link5/1(w_H_root) -> stateMachineFCN/10(r_sole_H_b), xCom1/2(w_H_b)
  Get Estimate/1 -> w_H_root_link4/1(qj), Debug/1(jointAngles), w_H_root_link5/1(qj), nu/1(qj), xCom/1(qj), stateMachineFCN/7(qj), holder 2/1, xCom1/1(qj), qj/1
  inertial/1 -> w_H_root_link4/2(inertial), Debug/2(inertial), w_H_root_link5/2(inertial)

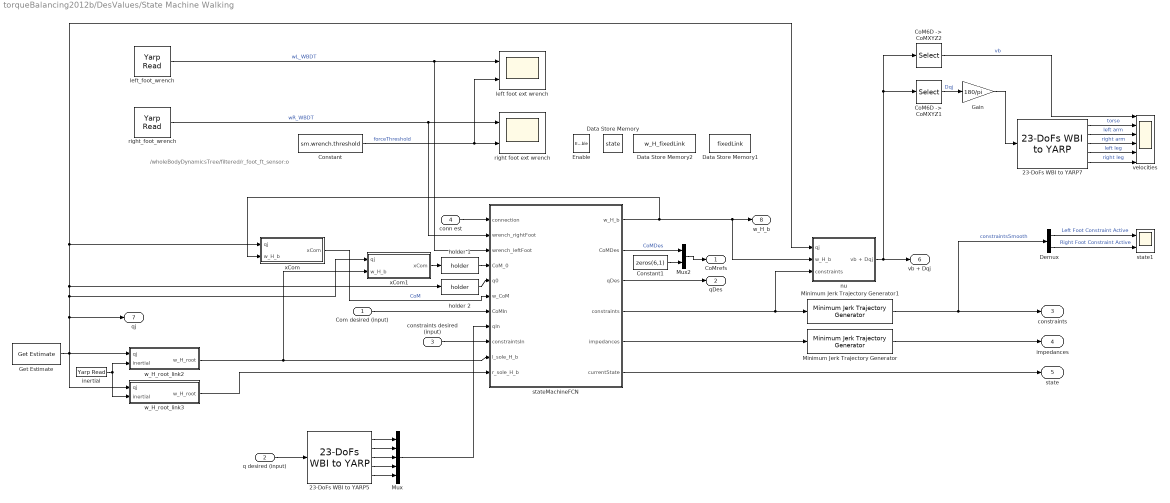
== system torqueBalancing2012b/DesValues/State Machine Walking ==
  note: /wholeBodyDynamicsTree/filtered/r_foot_ft_sensor:o
  Com desired (input) : Inport
  q desired (input) : Inport  Port=2
  constraints desired (input) : Inport  Port=3
  conn est : Inport  Port=4
  Enable : EnablePort
  23-DoFs WBI to YARP5 : WBToolboxLibrary/Utilities/23-DoFs WBI to YARP
  23-DoFs WBI to YARP7 : WBToolboxLibrary/Utilities/23-DoFs WBI to YARP
  "CoM6D ->  CoMXYZ1" : Selector  InputPortWidth=ROBOT_DOF+6  IndexOptions=Index vector (dialog)  Indices=[7:ROBOT_DOF+6]  OutputSizes=1
  "CoM6D ->  CoMXYZ2" : Selector  InputPortWidth=ROBOT_DOF+6  IndexOptions=Index vector (dialog)  Indices=[1 2 3 4 5 6]  OutputSizes=1
  Constant : Constant  Value=sm.wrench.threshold
  Constant1 : Constant  Value=zeros(6,1)
  Data Store Memory : DataStoreMemory  DataStoreName=state  InitialValue=sm.stateAt0  OutDataTypeStr=double
  Data Store Memory1 : DataStoreMemory  DataStoreName=fixedLink  InitialValue=1  OutDataTypeStr=double
  Data Store Memory2 : DataStoreMemory  DataStoreName=w_H_fixedLink  InitialValue=eye(4)  OutDataTypeStr=double
  Demux : Demux  Outputs=2
  Gain : Gain  Gain=180/pi
  Get Estimate : WBToolboxLibrary/wholeBodyStates/Get Estimate  estimateType=Joints Position  robotName=WBT_robotName  localName=WBT_modelName  wbiFile=WBT_wbiFilename  wbiList=WBT_wbiList
  Minimum Jerk Trajectory Generator : WBToolboxLibrary/Utilities/Minimum Jerk Trajectory Generator  externalSettlingTime=off  settlingTime=gain.SmoothingTimeImp  sampleTime=CONFIG.Ts  firstDerivatives=off  secondDerivatives=off  explicitInitialValue=off
  Minimum Jerk Trajectory Generator1 : WBToolboxLibrary/Utilities/Minimum Jerk Trajectory Generator  externalSettlingTime=off  settlingTime=smoothingTimeTransitionDynamics  sampleTime=CONFIG.Ts  firstDerivatives=off  secondDerivatives=off  explicitInitialValue=off
  Mux : Mux  Inputs=5
  Mux2 : Mux  Inputs=2
  holder 1 : WBToolboxLibrary/Utilities/holder 
  holder 2 : WBToolboxLibrary/Utilities/holder 
  inertial : WBToolboxLibrary/Utilities/Yarp Read  portName='/icub/inertial'  signalSize=12  blocking=off  timestamp=off  autoconnect=on  errorOnConnection=off
  left foot ext wrench : Scope  NumInputPorts=2
      settings: YMin=-49.77821~-5  YMax=218.07228~5
  left_foot_wrench : WBToolboxLibrary/Utilities/Yarp Read  portName='/wholeBodyDynamicsTree/left_leg/cartesianEndEffectorWrench:o'  signalSize=6  blocking=off  timestamp=off  autoconnect=on  errorOnConnection=off
  nu : Subsystem
  right foot ext wrench : Scope  NumInputPorts=2
      settings: ShowLegends=on  TimeRange=42.68  YMin=-145.04201~-5  YMax=387.7556~5
  right_foot_wrench : WBToolboxLibrary/Utilities/Yarp Read  portName='/wholeBodyDynamicsTree/right_leg/cartesianEndEffectorWrench:o'  signalSize=6  blocking=off  timestamp=off  autoconnect=on  errorOnConnection=off
  state1 : Scope  NumInputPorts=2
      settings: YMin=-0.14635~-5  YMax=1.12737~5  SaveName=ScopeData2
  stateMachineFCN : MATLAB Function  Priority=-1  TreatAsAtomicUnit=on
  velocities : Scope  NumInputPorts=6
      settings: YMin=-2.14738~-167.8498~-240.80577~-214.40022~-170.94682~-166.50539  YMax=2.60944~145.16937~76.88393~295.56172~218.42933~230.10458  SaveName=ScopeData2
  w_H_root_link2 : Subsystem  mask{link_name='l_sole'}
      mask prompts: link_name "link name"
      mask help:
      | This block evaluates the homogeneous transformation between the world and the root link, i.e. ^wH_b. It assumes that the link specified by the variable 'link_name' has a constant position
      | w.r.t. an inertial frame, but it can rotate arbitrarily. This rotation is retrived from the IMU sensor.
  w_H_root_link3 : Subsystem  mask{link_name='r_sole'}
      mask prompts: link_name "link name"
      mask help:
      | This block evaluates the homogeneous transformation between the world and the root link, i.e. ^wH_b. It assumes that the link specified by the variable 'link_name' has a constant position
      | w.r.t. an inertial frame, but it can rotate arbitrarily. This rotation is retrived from the IMU sensor.
  xCom : Subsystem  Priority=-2
  xCom1 : Subsystem  Priority=-2
  CoMrefs : Outport
  qDes : Outport  Port=2
  constraints : Outport  Port=3
  impedances : Outport  Port=4
  state : Outport  Port=5
  vb + Dqj : Outport  Port=6
  qj : Outport  Port=7
  w_H_b : Outport  Port=8
  wires:
  Constant/1 -> left foot ext wrench/2, right foot ext wrench/2  "forceThreshold"
  right_foot_wrench/1 -> right foot ext wrench/1, stateMachineFCN/2(wrench_rightFoot)  "wR_WBDT"
  xCom/1(xCom) -> stateMachineFCN/6(w_CoM)  "CoM"
  holder 2/1 -> stateMachineFCN/5(q0)
  stateMachineFCN/3(qDes) -> qDes/1
  stateMachineFCN/2(CoMDes) -> Mux2/1  "CoMDes"
  Mux2/1 -> CoMrefs/1
  Constant1/1 -> Mux2/2
  stateMachineFCN/5(impedances) -> Minimum Jerk Trajectory Generator/1
  stateMachineFCN/6(currentState) -> state/1
  Minimum Jerk Trajectory Generator1/1 -> Demux/1, constraints/1  "constraintsSmooth"
  stateMachineFCN/4(constraints) -> nu/3("constraints "), Minimum Jerk Trajectory Generator1/1
  Demux/1 -> state1/1  "Left Foot Constraint Active"
  Demux/2 -> state1/2  "Right Foot Constraint Active"
  left_foot_wrench/1 -> left foot ext wrench/1, stateMachineFCN/3(wrench_leftFoot)  "wL_WBDT"
  stateMachineFCN/1(w_H_b) -> xCom/2(w_H_b), nu/2(w_H_b), w_H_b/1
  nu/1(vb + Dqj) -> vb + Dqj/1, "CoM6D ->  CoMXYZ1"/1, "CoM6D ->  CoMXYZ2"/1
  Minimum Jerk Trajectory Generator/1 -> impedances/1
  "CoM6D ->  CoMXYZ2"/1 -> velocities/1  "vb"
  "CoM6D ->  CoMXYZ1"/1 -> Gain/1  "Dqj"
  23-DoFs WBI to YARP7/1 -> velocities/2  "torso"
  23-DoFs WBI to YARP7/2 -> velocities/3  "left arm"
  23-DoFs WBI to YARP7/3 -> velocities/4  "right arm"
  23-DoFs WBI to YARP7/4 -> velocities/5  "left leg"
  23-DoFs WBI to YARP7/5 -> velocities/6  "right leg"
  Gain/1 -> 23-DoFs WBI to YARP7/1
  w_H_root_link2/1(w_H_root) -> stateMachineFCN/10(l_sole_H_b), xCom1/2(w_H_b)
  w_H_root_link3/1(w_H_root) -> stateMachineFCN/11(r_sole_H_b)
  Get Estimate/1 -> nu/1(qj), xCom/1(qj), holder 2/1, xCom1/1(qj), qj/1, w_H_root_link2/1(qj), w_H_root_link3/1(qj)
  inertial/1 -> w_H_root_link2/2(inertial), w_H_root_link3/2(inertial)
  Com desired (input)/1 -> stateMachineFCN/7(CoMIn)
  constraints desired (input)/1 -> stateMachineFCN/9(constraintsIn)
  holder 1/1 -> stateMachineFCN/4(CoM_0)
  xCom1/1(xCom) -> holder 1/1
  conn est/1 -> stateMachineFCN/1(connection)
  q desired (input)/1 -> 23-DoFs WBI to YARP5/1
  23-DoFs WBI to YARP5/5 -> Mux/5
  23-DoFs WBI to YARP5/3 -> Mux/3
  23-DoFs WBI to YARP5/2 -> Mux/2
  23-DoFs WBI to YARP5/4 -> Mux/4
  23-DoFs WBI to YARP5/1 -> Mux/1
  Mux/1 -> stateMachineFCN/8(qIn)

== system torqueBalancing2012b/DesValues/Subsystem ==
  conn status 1 : Inport
  conn status 2 : Inport  Port=2
  conn status 3 : Inport  Port=3
  Compare To Zero3 : simulink/Logic and Bit Operations/Compare To Zero  relop=>  OutDataTypeStr=boolean
  Compare To Zero4 : simulink/Logic and Bit Operations/Compare To Zero  relop=>  OutDataTypeStr=boolean
  Compare To Zero5 : simulink/Logic and Bit Operations/Compare To Zero  relop=>  OutDataTypeStr=boolean
  Logical Operator : Logic  Inputs=3  AllPortsSameDT=off  OutDataTypeStr=boolean
  connection check : Outport
  wires:
  Logical Operator/1 -> connection check/1
  Compare To Zero4/1 -> Logical Operator/3
  conn status 1/1 -> Compare To Zero3/1
  Compare To Zero3/1 -> Logical Operator/1
  conn status 3/1 -> Compare To Zero4/1
  Compare To Zero5/1 -> Logical Operator/2
  conn status 2/1 -> Compare To Zero5/1

== system torqueBalancing2012b/DesValues/Visualize hom transf4 ==
  H : Inport
  upBase : Inport  Port=2
  "CoM6D ->  CoMXYZ1" : Selector  NumberOfDimensions=2  InputPortWidth=7  IndexOptions=Index vector (dialog),Index vector (dialog)  Indices=[1 2 3],[1 2 3]  OutputSizes=1,1
  "CoM6D ->  CoMXYZ2" : Selector  NumberOfDimensions=2  InputPortWidth=7  IndexOptions=Index vector (dialog),Index vector (dialog)  Indices=[1 2 3],[4]  OutputSizes=1,1
  Hom : Scope  NumInputPorts=2
      settings: ShowLegends=on  YMin=-1.25~-0.125  YMax=1.25~1.125  SaveName=ScopeData3
  R : Scope  NumInputPorts=2
      settings: YMin=-0.09594~-0.125  YMax=0.20308~1.125
  p : Scope  NumInputPorts=2
      settings: YMin=-1.00000~-0.125  YMax=1.00000~1.125  SaveName=ScopeData2
  wires:
  "CoM6D ->  CoMXYZ1"/1 -> R/1
  "CoM6D ->  CoMXYZ2"/1 -> p/1
  H/1 -> "CoM6D ->  CoMXYZ2"/1, Hom/1, "CoM6D ->  CoMXYZ1"/1
  upBase/1 -> p/2, R/2, Hom/2

== system torqueBalancing2012b/DesValues/centroidalOrient_partialDer ==
  qDes : Inport
  qj : Inport  Port=2
  Jc0 : Subsystem
  Jw0_base : Subsystem
  Jw0_joints : Subsystem
  generate Jw0 : MATLAB Function  TreatAsAtomicUnit=on
  l_sole_H_root_link : Subsystem
  deltaphi_old : Outport
  wires:
  generate Jw0/1(Deltaphi) -> deltaphi_old/1
  l_sole_H_root_link/1(W_H_B0) -> Jc0/1(W_H_b0), Jw0_joints/1(W_H_b0), Jw0_base/1(W_H_b0)
  qDes/1 -> generate Jw0/5(qj0), l_sole_H_root_link/1(qjDes), Jw0_base/2(qjDes), Jw0_joints/2(qjDes), Jc0/2(qjDes)
  Jw0_base/1(Jw0b) -> generate Jw0/1(Jw0b)
  Jw0_joints/1(Jw0j) -> generate Jw0/2(Jw0j)
  Jc0/1(Jc0) -> generate Jw0/3(Jc0)
  qj/1 -> generate Jw0/4(qj)

== system torqueBalancing2012b/DesValues/centroidalOrient_partialDer_at_0 ==
  qjDes : Inport
  qj : Inport  Port=2
  Centroidal Momentum2 : WBToolboxLibrary/wholeBodyModel/Dynamics/Centroidal Momentum  robotName=WBT_robotName  localName=WBT_modelName  wbiFile=WBT_wbiFilename  wbiList=WBT_wbiList
  Demux : Demux  Outputs=[3;3]
  Jacobian_Lfoot : WBToolboxLibrary/wholeBodyModel/Jacobians/Jacobian  frameName='l_sole'  robotName=WBT_robotName  localName=WBT_modelName  wbiFile=WBT_wbiFilename  wbiList=WBT_wbiList
  MATLAB Function : MATLAB Function  TreatAsAtomicUnit=on
  Sum : Sum  Inputs=|-+
  Terminator : Terminator
  l_sole_H_root_link : Subsystem
  Deltaphi : Outport
  wires:
  Demux/2 -> Deltaphi/1
  qjDes/1 -> Jacobian_Lfoot/2, Sum/1, Centroidal Momentum2/2, l_sole_H_root_link/1(qjDes)
  l_sole_H_root_link/1(W_H_b0) -> Centroidal Momentum2/1, Jacobian_Lfoot/1
  Jacobian_Lfoot/1 -> MATLAB Function/1(Jclf)
  Sum/1 -> Centroidal Momentum2/4, MATLAB Function/2(Deltaqj)
  MATLAB Function/1(vbar) -> Centroidal Momentum2/3
  qj/1 -> Sum/2
  Demux/1 -> Terminator/1
  Centroidal Momentum2/1 -> Demux/1

== system torqueBalancing2012b/DesValues/nonlinearImpedances ==
  qMin : Inport
  qMax : Inport  Port=2
  qDes : Inport  Port=3
  q : Inport  Port=4
  23-DoFs WBI to YARP2 : WBCLibrary/Utilities/23-DoFs WBI to YARP  Commented=on
  Saturation2 : Saturate  Commented=on  UpperLimit=impedencesSat(1)  LowerLimit=0  SampleTime=Ts
  Saturation3 : Saturate  Commented=on  UpperLimit=impedencesSat(2)  LowerLimit=0  SampleTime=Ts
  Saturation4 : Saturate  Commented=on  UpperLimit=impedencesSat(2)  LowerLimit=0  SampleTime=Ts
  Saturation5 : Saturate  Commented=on  UpperLimit=impedencesSat(3)  LowerLimit=0  SampleTime=Ts
  Saturation6 : Saturate  Commented=on  UpperLimit=impedencesSat(3)  LowerLimit=0  SampleTime=Ts
  nonlinearImpedances : Scope  Commented=on  NumInputPorts=5
      settings: ShowLegends=on  TimeRange=25  YMin=-50~-50~-50~0~0  YMax=50~50~50~1000~1000
  nonlinearImpedances1 : Scope  Commented=on
      settings: ShowLegends=on  TimeRange=25  YMin=-50  YMax=50
  "nonlinearPosturalGains " : MATLAB Function  TreatAsAtomicUnit=on
  yarp to WBI : WBCLibrary/Utilities/yarp to WBI  Commented=on
  nonLinSatImp : Outport
  wires:
  23-DoFs WBI to YARP2/1 -> Saturation2/1
  23-DoFs WBI to YARP2/2 -> Saturation3/1
  23-DoFs WBI to YARP2/3 -> Saturation4/1
  23-DoFs WBI to YARP2/5 -> Saturation6/1
  "nonlinearPosturalGains "/1(nonlinearImpedences) -> nonlinearImpedances1/1, nonLinSatImp/1, 23-DoFs WBI to YARP2/1
  qMin/1 -> "nonlinearPosturalGains "/3(qMin)
  qMax/1 -> "nonlinearPosturalGains "/4(qMax)
  q/1 -> "nonlinearPosturalGains "/2(q)
  Saturation6/1 -> nonlinearImpedances/5, yarp to WBI/5  "rightLeg"
  Saturation4/1 -> nonlinearImpedances/3, yarp to WBI/3  "rightArm"
  Saturation5/1 -> nonlinearImpedances/4, yarp to WBI/4  "leftLeg"
  Saturation3/1 -> nonlinearImpedances/2, yarp to WBI/2  "leftArm"
  Saturation2/1 -> nonlinearImpedances/1, yarp to WBI/1  "torso"
  23-DoFs WBI to YARP2/4 -> Saturation5/1
  qDes/1 -> "nonlinearPosturalGains "/1(qDes)

== system torqueBalancing2012b/Dump and visualize/ZMPs ==
  fDesQP : Inport
  Demux1 : Demux  Outputs=3
  Demux2 : Demux  Outputs=3
  Divide{4..7} (4 alike) : Product  Inputs=*/
  Gain3 : Gain  Gain=-1
  Gain4 : Gain  Gain=-1
  Mux : Mux  Inputs=2
  Mux1 : Mux  Inputs=2
  fz taux tauy Left : Selector  InputPortWidth=12  IndexOptions=Index vector (dialog)  Indices=[3 4 5]  OutputSizes=1
  fz taux tauy Right : Selector  InputPortWidth=12  IndexOptions=Index vector (dialog)  Indices=[9 10 11]  OutputSizes=1
  ZMP_LeftFoot : Outport
  ZMP_RightFoot : Outport  Port=2
  wires:
  fz taux tauy Left/1 -> Demux1/1
  Demux1/1 -> Divide4/2, Divide5/2
  Divide7/1 -> Gain4/1
  Divide4/1 -> Mux/2
  Divide5/1 -> Gain3/1
  fz taux tauy Right/1 -> Demux2/1
  Demux2/1 -> Divide6/2, Divide7/2
  fDesQP/1 -> fz taux tauy Left/1, fz taux tauy Right/1
  Gain3/1 -> Mux/1
  Mux/1 -> ZMP_LeftFoot/1
  Divide6/1 -> Mux1/2
  Gain4/1 -> Mux1/1
  Mux1/1 -> ZMP_RightFoot/1
  Demux1/2 -> Divide4/1  "tauxL"
  Demux1/3 -> Divide5/1  "tauyL"
  Demux2/2 -> Divide6/1  "tauxR"
  Demux2/3 -> Divide7/1  "tauyR"

== system torqueBalancing2012b/Dump and visualize/plotNorms ==
  qTile_LeftLeg : Inport
  qTile_RightLeg : Inport  Port=2
  Constant : Constant  Value=sm.joints.thresholdInContact
  Constant1 : Constant  Value=sm.joints.thresholdInContact
  Constant2 : Constant  Value=sm.joints.thresholdNotInContact
  Constant3 : Constant  Value=sm.joints.thresholdNotInContact
  Mux : Mux  Inputs=3
  Mux1 : Mux  Inputs=3
  norm : MATLAB Function  TreatAsAtomicUnit=on
  norm(qTilde) : Scope  NumInputPorts=2
      settings: ShowLegends=on  YMin=-6.25~-6.25  YMax=56.25~56.25
  norm1 : MATLAB Function  TreatAsAtomicUnit=on
  wires:
  Constant/1 -> Mux/2  "thresholdLL"
  qTile_LeftLeg/1 -> norm1/1(u)
  qTile_RightLeg/1 -> norm/1(u)
  norm/1(normU) -> Mux1/1  "norm(qTilde_RightL)"
  norm1/1(normU) -> Mux/1  "norm(qTilde_LeftL)"
  Mux/1 -> norm(qTilde)/1
  Mux1/1 -> norm(qTilde)/2
  Constant2/1 -> Mux/3
  Constant1/1 -> Mux1/2
  Constant3/1 -> Mux1/3

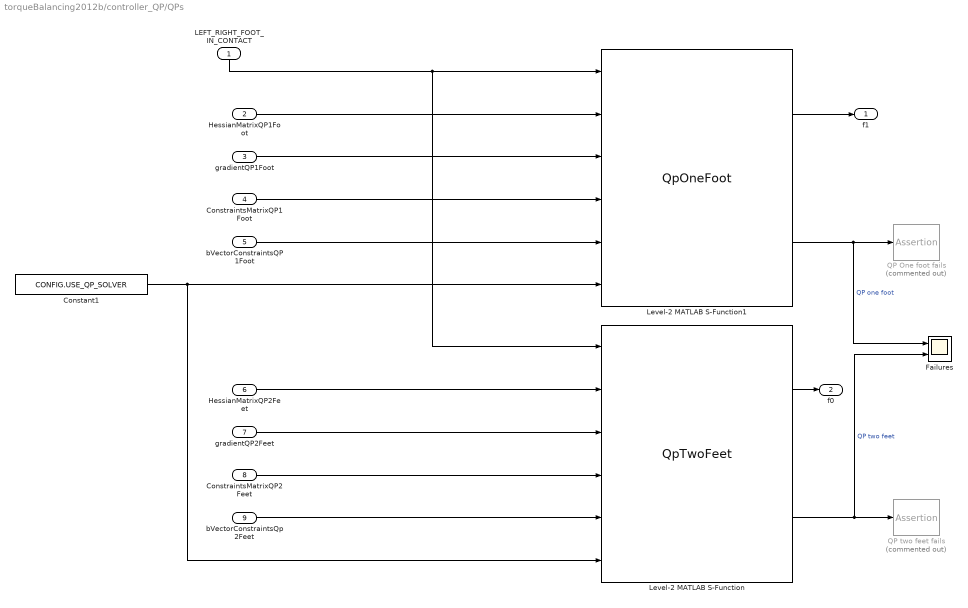
== system torqueBalancing2012b/controller_QP/QPs ==
  LEFT_RIGHT_FOOT_IN_CONTACT : Inport
  HessianMatrixQP1Foot : Inport  Port=2
  gradientQP1Foot : Inport  Port=3
  ConstraintsMatrixQP1Foot : Inport  Port=4
  bVectorConstraintsQP1Foot : Inport  Port=5
  HessianMatrixQP2Feet : Inport  Port=6
  gradientQP2Feet : Inport  Port=7
  ConstraintsMatrixQP2Feet : Inport  Port=8
  bVectorConstraintsQp2Feet : Inport  Port=9
  Constant1 : Constant  Value=CONFIG.USE_QP_SOLVER
  Failures : Scope  NumInputPorts=2
      settings: YMin=-1.00000~-1.00000  YMax=1.00000~1.00000
  Level-2 MATLAB S-Function : M-S-Function  FunctionName=QpTwoFeet
  Level-2 MATLAB S-Function1 : M-S-Function  FunctionName=QpOneFoot
  QP One foot fails : Assertion  Commented=on  Enabled=on
  QP two feet fails : Assertion  Commented=on  Enabled=on
  f1 : Outport
  f0 : Outport  Port=2
  wires:
  LEFT_RIGHT_FOOT_IN_CONTACT/1 -> Level-2 MATLAB S-Function1/1, Level-2 MATLAB S-Function/1
  gradientQP2Feet/1 -> Level-2 MATLAB S-Function/3
  HessianMatrixQP1Foot/1 -> Level-2 MATLAB S-Function1/2
  ConstraintsMatrixQP2Feet/1 -> Level-2 MATLAB S-Function/4
  gradientQP1Foot/1 -> Level-2 MATLAB S-Function1/3
  HessianMatrixQP2Feet/1 -> Level-2 MATLAB S-Function/2
  Level-2 MATLAB S-Function/1 -> f0/1
  bVectorConstraintsQp2Feet/1 -> Level-2 MATLAB S-Function/5
  Level-2 MATLAB S-Function1/1 -> f1/1
  ConstraintsMatrixQP1Foot/1 -> Level-2 MATLAB S-Function1/4
  bVectorConstraintsQP1Foot/1 -> Level-2 MATLAB S-Function1/5
  Level-2 MATLAB S-Function/2 -> Failures/2, QP two feet fails/1  "QP two feet"
  Constant1/1 -> Level-2 MATLAB S-Function/6, Level-2 MATLAB S-Function1/6
  Level-2 MATLAB S-Function1/2 -> Failures/1, QP One foot fails/1  "QP one foot"

== system torqueBalancing2012b/controller_QP/xCom ==
  w_H_b : Inport
  qj : Inport  Port=2
  "CoM6D ->  CoMXYZ2" : Selector  NumberOfDimensions=2  InputPortWidth=7  IndexOptions=Index vector (dialog),Index vector (dialog)  Indices=[1 2 3],[4]  OutputSizes=1,1
  com : WBToolboxLibrary/wholeBodyModel/Kinematics/Forward Kinematics  frameName='com'  robotName=WBT_robotName  localName=WBT_modelName  wbiFile=WBT_wbiFilename  wbiList=WBT_wbiList
  xCom : Outport
  wires:
  qj/1 -> com/2
  "CoM6D ->  CoMXYZ2"/1 -> xCom/1
  com/1 -> "CoM6D ->  CoMXYZ2"/1
  w_H_b/1 -> com/1
